simulink model "practica2c"  (R2022a)
settings: Solver=FixedStepAuto  StartTime=0.0  StopTime=10.0  RelTol=1e-3  EnableMultiTasking=on
undefined symbols (not defined in the file): ni, P, ref, sens, t_sim
libraries: legoev3lib x6, simulink x1
settings Model: ExtModeTrigDuration=2  Creator=marcos  LastModifiedBy=Sersa
settings SolverCC: AlgebraicLoopSolver=TrustRegion  PositivePriorityOrder=on
settings OptimizationCC: EnhancedBackFolding=on  PassReuseOutputArgsAs=Individual arguments  ZeroExternalMemoryAtStartup=off  ZeroInternalMemoryAtStartup=off  MaxStackSize=64  OptimizeBlockOrder=speed  DifferentSizesBufferReuse=on  OptimizationCustomize=off  EfficientTunableParamExpr=on
settings DebuggingCC: ParameterTunabilityLossMsg=error  UnconnectedInputMsg=warning  UnconnectedOutputMsg=warning  UnconnectedLineMsg=warning
settings HardwareCC: ProdBitPerPointer=32  ProdBitPerSizeT=32  ProdBitPerPtrDiffT=32  ProdLargestAtomicInteger=Long  ProdWordSize=32  ProdHWDeviceType=ARM Compatible->ARM 9
settings SFSimCC: MATLABDynamicMemAlloc=off
settings RTWCC: SystemTargetFile=ert.tlc  HardwareBoard=LEGO MINDSTORMS EV3  TLCOptions="-aInlineSetEventsForThisBaseRateFcn=TLC_FALSE -aSuppressMultiTaskScheduler=TLC_FALSE  -aRateBasedStepFcn=0"  TemplateMakefile=ert_default_tmf  GenerateReport=on  Toolchain=Sourcery G++ Lite v2009q3  IncludeHyperlinkInReport=on  LaunchReport=on  GenerateTraceInfo=on  GenerateTraceReport=on  GenerateTraceReportSl=on  GenerateTraceReportSf=on  GenerateTraceReportEml=on
settings CodeAppCC: ForceParamTrailComments=on  IgnoreCustomStorageClasses=off  OperatorAnnotations=on  SimulinkDataObjDesc=on  SFDataObjDesc=on  InsertBlockDesc=on
settings ERTTargetCC: SupportContinuousTime=on  SupportVariableSizeSignals=on

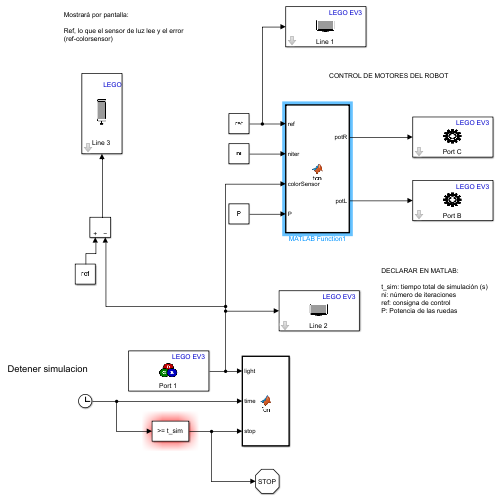
[thumbnail: Simulink's stored preview of the top-level diagram]
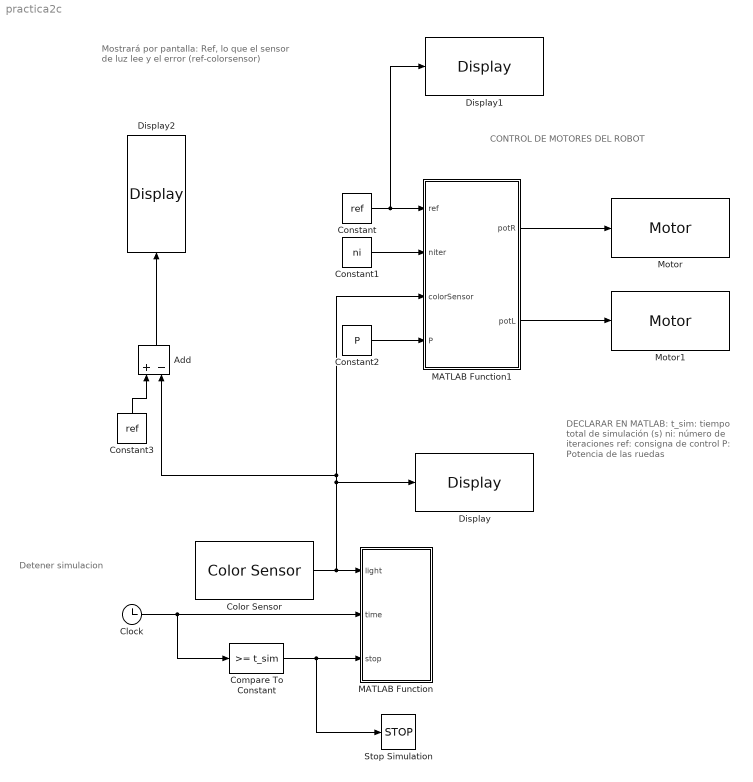
== system practica2c ==
  note: Mostrará por pantalla:
      |
      | Ref, lo que el sensor de luz lee y el error
      | (ref-colorsensor)
  note: CONTROL DE MOTORES DEL ROBOT
  note: DECLARAR EN MATLAB:
      |
      | t_sim: tiempo total de simulación (s)
      | ni: número de iteraciones
      | ref: consigna de control
      | P: Potencia de las ruedas
  note: Detener simulacion
  Add : Sum  Inputs=+-
  Clock : Clock
  Color Sensor : legoev3lib/Color Sensor  portNumber=1  mode=Reflected light intensity  sampleTime=0.1
      settings: SourceProductBaseCode=LEGOEV3
  Compare To Constant : simulink/Logic and Bit Operations/Compare To Constant  relop=>=  const=t_sim  OutDataTypeStr=boolean
  Constant : Constant  Value=ref
  Constant1 : Constant  Value=ni
  Constant2 : Constant  Value=P
  Constant3 : Constant  Value=ref
  Display : legoev3lib/Display  slcdStr=sens:  slcdLine=2  slcdFormat=Decimal
      settings: SourceProductBaseCode=LEGOEV3
  Display1 : legoev3lib/Display  slcdStr=ref=  slcdLine=1  slcdFormat=Decimal
      settings: SourceProductBaseCode=LEGOEV3
  Display2 : legoev3lib/Display  slcdStr=error:  slcdLine=3  slcdFormat=Decimal
      settings: SourceProductBaseCode=LEGOEV3
  MATLAB Function : MATLAB Function  TreatAsAtomicUnit=on
  MATLAB Function1 : MATLAB Function  TreatAsAtomicUnit=on
  Motor : legoev3lib/Motor  sportNumber=C  sstopAction=Brake
  Motor1 : legoev3lib/Motor  sportNumber=B  sstopAction=Brake
  Stop Simulation : Stop
  wires:
  Clock/1 -> Compare To Constant/1, MATLAB Function/2(time)
  Compare To Constant/1 -> Stop Simulation/1, MATLAB Function/3(stop)
  Constant1/1 -> MATLAB Function1/2(niter)
  Constant/1 -> Display1/1, MATLAB Function1/1(ref)
  MATLAB Function1/1(potR) -> Motor/1
  MATLAB Function1/2(potL) -> Motor1/1
  Constant2/1 -> MATLAB Function1/4(P)
  Add/1 -> Display2/1
  Constant3/1 -> Add/1
  Color Sensor/1 -> MATLAB Function/1(light), Display/1, Add/2, MATLAB Function1/3(colorSensor)

== matlab function practica2c/MATLAB Function1 ==
  data: ref input; potR output; niter input; colorSensor input; potL output; P input
function [potR,potL]    = fcn(ref,niter,colorSensor,P)
    persistent iter;
    
    if (isempty(iter))
        iter = 0;
    end
    
    iter = iter +1;
    colorSensor = int32(colorSensor);
    
    if(iter <= niter)
    %Calculo del error

         err = ref-colorSensor;
        
        %Capa la potencia de cada rueda. error debería de acercarse lo
        %máximo posible a 0, que es cuando la potencia será P. En caso de
        %ser mayor que 5 o menor que -5 se parará para corregir la
        %alineación
        if(err>5)
            potR = int32(-P);
            potL = int32(P);
        elseif (err<=-5)
            potR = int32(P);
            potL = int32(-P);
        else
            potR = int32(P);
            potL = int32(P);

        end   
    else
        potR =int32(0);
        potL =int32(0);
    end

== matlab function practica2c/MATLAB Function ==
  data: light input; time input; stop input
function fcn(light, time, stop)

persistent myFile;

if (isempty(myFile))
    myFile = fopen('D:\mylog.txt','w');
end

if (myFile >= 0)
    if (stop > 0)
        fclose(myFile);
        myFile = -1;
    else
        fprintf(myFile, '%f\t%i\n', time, int32(light));
    end
end
